simulink model "NM100A_MotVelCtrl"  (R2013b)
settings: Solver=FixedStepDiscrete  SolverMode=SingleTasking  StartTime=0.0  StopTime=1  FixedStep=0.002  RelTol=1e-3
values from neighbouring files (symbols this model uses):
  ARCHGLBPRM_2MILLISEC_SEC_F32 = DataDict.Constant    [NM100A_MotVelCtrl_DataDict.m]
  DERIVTVLPFILTICONLOWRLIM_SEC_F32 = DataDict.Constant    [NM100A_MotVelCtrl_DataDict.m]
  FALSE_CNT_LGC = DataDict.Constant    [NM100A_MotVelCtrl_DataDict.m]
  MOTVELTHDRAMPDWNCMPL_MOTRADPERSEC_F32 = DataDict.Constant    [NM100A_MotVelCtrl_DataDict.m]
  ONEMILLISEC_SEC_F32 = DataDict.Constant    [NM100A_MotVelCtrl_DataDict.m]
  TITHDRAMPDWNCMPL_CNT_U16 = DataDict.Constant    [NM100A_MotVelCtrl_DataDict.m]
  TRUE_CNT_LGC = DataDict.Constant    [NM100A_MotVelCtrl_DataDict.m]
  ZEROMOTVELTAR_MOTRADPERSEC_F32 = DataDict.Constant    [NM100A_MotVelCtrl_DataDict.m]
  ZEROTQCMD_MOTNWTMTR_F32 = DataDict.Constant    [NM100A_MotVelCtrl_DataDict.m]
libraries: NxtrLim x13, simulink x1, NxtrAbslt x1, NxtrMax x1
(part 3 of 4)

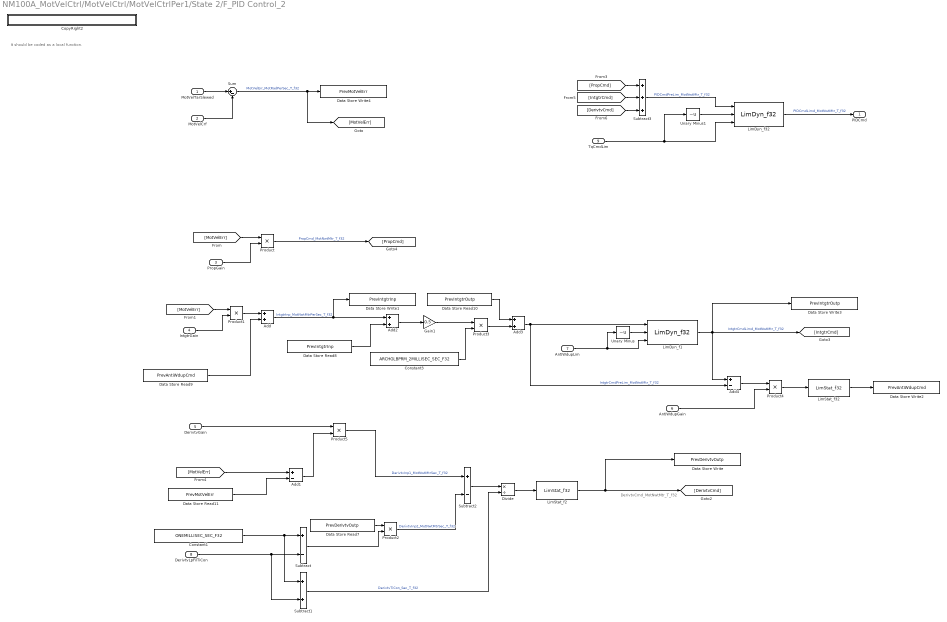
== system NM100A_MotVelCtrl/MotVelCtrl/MotVelCtrlPer1/State 2/F_PID Control_2 ==
  note: DerivtvCmd_MotNwtMtr_T_f32
  note: It should be coded as a local function.
  MotVelTarSlewed : Inport  RequirementInfo="{'linktype_rmi_doors' '00010020 (/E-STEER Core/SubSystem Specifications/Manufacturing Service/NM100A_Motor Velocity Control Function Requirement)' '#NM100A_30' 'true' 'REQ:  NM100A_30' '' } %GIDa_110524b8_0db1_43e8_8f08_01f20704c4bb"
  MotVelCrf : Inport  RequirementInfo="{'linktype_rmi_doors' '00010020 (/E-STEER Core/SubSystem Specifications/Manufacturing Service/NM100A_Motor Velocity Control Function Requirement)' '#NM100A_30' 'true' 'REQ:  NM100A_30' '' } %GIDa_7d766da7_5e04_40ea_badd_d72d93f3cd8f"  Port=2
  PropGain : Inport  RequirementInfo="{'linktype_rmi_doors' '00010020 (/E-STEER Core/SubSystem Specifications/Manufacturing Service/NM100A_Motor Velocity Control Function Requirement)' '#NM100A_112' 'true' 'REQ:  NM100A_112' '' } %GIDa_a1a22dbd_d264_4c62_8ca1_990479f3e1bd"  Port=3
  IntgtrGain : Inport  RequirementInfo="{'linktype_rmi_doors' '00010020 (/E-STEER Core/SubSystem Specifications/Manufacturing Service/NM100A_Motor Velocity Control Function Requirement)' '#NM100A_115' 'true' 'REQ:  NM100A_115' '' } %GIDa_1390f88b_fe28_4670_9b5c_e6d73974c688"  Port=4
  DerivtvGain : Inport  RequirementInfo="{'linktype_rmi_doors' '00010020 (/E-STEER Core/SubSystem Specifications/Manufacturing Service/NM100A_Motor Velocity Control Function Requirement)' '#NM100A_116' 'true' 'REQ:  NM100A_116' '' } %GIDa_f6cc3c77_9957_4476_a97a_fb14260ee4dc"  Port=5
  AntiWdupGain : Inport  RequirementInfo="{'linktype_rmi_doors' '00010020 (/E-STEER Core/SubSystem Specifications/Manufacturing Service/NM100A_Motor Velocity Control Function Requirement)' '#NM100A_118' 'true' 'REQ:  NM100A_118' '' } %GIDa_56666803_4490_41e6_aeb7_9ef0196ec25d"  Port=6
  AntiWdupLim : Inport  RequirementInfo="{'linktype_rmi_doors' '00010020 (/E-STEER Core/SubSystem Specifications/Manufacturing Service/NM100A_Motor Velocity Control Function Requirement)' '#NM100A_118' 'true' 'REQ:  NM100A_118' '' } %GIDa_11bba2b0_a075_4aca_bc0b_995865d16d8e"  Port=7
  DerivtvLpFilTiCon : Inport  RequirementInfo="{'linktype_rmi_doors' '00010020 (/E-STEER Core/SubSystem Specifications/Manufacturing Service/NM100A_Motor Velocity Control Function Requirement)' '#NM100A_116' 'true' 'REQ:  NM100A_116' '' } %GIDa_2802fec0_4346_4fda_bccf_964533d4d2f8"  Port=8
  TqCmdLim : Inport  RequirementInfo="{'linktype_rmi_doors' '00010020 (/E-STEER Core/SubSystem Specifications/Manufacturing Service/NM100A_Motor Velocity Control Function Requirement)' '#NM100A_123' 'true' 'REQ:  NM100A_123' '' } %GIDa_855cb0b5_ed49_433d_978f_0dace05c254b"  Port=9
  Add : Sum  RequirementInfo="{'linktype_rmi_doors' '00010020 (/E-STEER Core/SubSystem Specifications/Manufacturing Service/NM100A_Motor Velocity Control Function Requirement)' '#NM100A_115' 'true' 'REQ:  NM100A_115' '' } %GIDa_6815d85c_18d2_448a_90c3_eea3a5c7f45e"
  Add1 : Sum  RequirementInfo="{'linktype_rmi_doors' '00010020 (/E-STEER Core/SubSystem Specifications/Manufacturing Service/NM100A_Motor Velocity Control Function Requirement)' '#NM100A_116' 'true' 'REQ:  NM100A_116' '' } %GIDa_f4b28a13_3ee6_406c_9849_7eac37b89283"  Inputs=+-
  Add2 : Sum  RequirementInfo="{'linktype_rmi_doors' '00010020 (/E-STEER Core/SubSystem Specifications/Manufacturing Service/NM100A_Motor Velocity Control Function Requirement)' '#NM100A_115' 'true' 'REQ:  NM100A_115' '' } %GIDa_9422ee42_1d4f_4bea_b4bf_ebe76635d43d"
  Add3 : Sum  RequirementInfo="{'linktype_rmi_doors' '00010020 (/E-STEER Core/SubSystem Specifications/Manufacturing Service/NM100A_Motor Velocity Control Function Requirement)' '#NM100A_115' 'true' 'REQ:  NM100A_115' '' } %GIDa_cc936411_c916_404a_ab30_f6a397637365"
  Add4 : Sum  RequirementInfo={'linktype_rmi_doors' '00010020 (/E-STEER Core/SubSystem Specifications/Manufacturing Service/NM100A_Motor Velocity Control Function Requirement)' '#NM100A_118' 'true' 'REQ:NM100A_118' '' } %GIDa_b21f0add_36e5_418f_9ceb_17b3d59b7e90  Inputs=+-
  Constant1 : Constant  RequirementInfo="{'linktype_rmi_doors' '00010020 (/E-STEER Core/SubSystem Specifications/Manufacturing Service/NM100A_Motor Velocity Control Function Requirement)' '#NM100A_116' 'true' 'REQ:  NM100A_116' '' } %GIDa_f3e2cce3_6137_4c8a_aa56_8064cca81233"  Value=ONEMILLISEC_SEC_F32
  Constant3 : Constant  RequirementInfo="{'linktype_rmi_doors' '00010020 (/E-STEER Core/SubSystem Specifications/Manufacturing Service/NM100A_Motor Velocity Control Function Requirement)' '#NM100A_115' 'true' 'REQ:  NM100A_115' '' } %GIDa_c43bbe87_f3ae_4efd_b0d8_54889718fd03"  Value=ARCHGLBPRM_2MILLISEC_SEC_F32
  CopyRight2 : Subsystem  Description=|  mask(Copyright Information){none=on}
      | Copyright info block.                                               
      |                                                                     
      | Place copyright information at the top of every subsystem in design.
      mask prompts: none "No parameters"
      mask help: Place copyright information at the top of every subsystem in design.
      mask Display:
      | NxtrConf = 'Nexteer Confidential';
      | 
      | sys = bdroot; %handle for the current model ("system")
      | first = get_param(sys,'Created');
      | if(isempty(first))
      |     first = datestr(now,'yyyy');
      | else
      |     first = first(end-3:end);  %year is last four digits
      | end
      | 
      | last = get_param(sys,'LastModifiedDate');
      | if isempty(last)
      |     last = datestr(now,'yyyy');
      | else
      |     last = last(end-3:end);
      | end
      | 
      | if strcmp(first,last)
      |     fprintf('%s -- Copyright %s Nexteer',NxtrConf,first)
      | else
      |     fprintf('%s -- %s%s- %s Nexteer',NxtrConf,char(169),first,last)
      | end
  Data Store Read10 : DataStoreRead  RequirementInfo="{'linktype_rmi_doors' '00010020 (/E-STEER Core/SubSystem Specifications/Manufacturing Service/NM100A_Motor Velocity Control Function Requirement)' '#NM100A_115' 'true' 'REQ:  NM100A_115' '' } %GIDa_57049909_113a_42ec_bae6_d87ca5e4f12b"  Priority=1  DataStoreName=PrevIntgtrOutp
  Data Store Read11 : DataStoreRead  RequirementInfo="{'linktype_rmi_doors' '00010020 (/E-STEER Core/SubSystem Specifications/Manufacturing Service/NM100A_Motor Velocity Control Function Requirement)' '#NM100A_116' 'true' 'REQ:  NM100A_116' '' } %GIDa_9f5ca0ec_ed47_41b3_b6b4_071471159927"  Priority=1  DataStoreName=PrevMotVelErr
  Data Store Read7 : DataStoreRead  RequirementInfo="{'linktype_rmi_doors' '00010020 (/E-STEER Core/SubSystem Specifications/Manufacturing Service/NM100A_Motor Velocity Control Function Requirement)' '#NM100A_116' 'true' 'REQ:  NM100A_116' '' } %GIDa_6db4a11a_7baf_4ed8_9c4d_f159cd772cec"  Priority=1  DataStoreName=PrevDerivtvOutp
  Data Store Read8 : DataStoreRead  RequirementInfo="{'linktype_rmi_doors' '00010020 (/E-STEER Core/SubSystem Specifications/Manufacturing Service/NM100A_Motor Velocity Control Function Requirement)' '#NM100A_115' 'true' 'REQ:  NM100A_115' '' } %GIDa_7cb75691_c32e_45f7_8fbd_fb2078527a41"  Priority=1  DataStoreName=PrevIntgtrInp
  Data Store Read9 : DataStoreRead  RequirementInfo="{'linktype_rmi_doors' '00010020 (/E-STEER Core/SubSystem Specifications/Manufacturing Service/NM100A_Motor Velocity Control Function Requirement)' '#NM100A_118' 'true' 'REQ:  NM100A_118' '' } %GIDa_fca8d963_6714_4519_b1fa_d800b04f6915"  Priority=1  DataStoreName=PrevAntiWdupCmd
  Data Store Write : DataStoreWrite  RequirementInfo="{'linktype_rmi_doors' '00010020 (/E-STEER Core/SubSystem Specifications/Manufacturing Service/NM100A_Motor Velocity Control Function Requirement)' '#NM100A_116' 'true' 'REQ:  NM100A_116' '' } %GIDa_c8470beb_41bb_4bfc_8c04_56d815b5965f"  Priority=2  DataStoreName=PrevDerivtvOutp
  Data Store Write1 : DataStoreWrite  RequirementInfo="{'linktype_rmi_doors' '00010020 (/E-STEER Core/SubSystem Specifications/Manufacturing Service/NM100A_Motor Velocity Control Function Requirement)' '#NM100A_115' 'true' 'REQ:  NM100A_115' '' } %GIDa_ba0b9b43_91f2_4915_a3e9_835597968f46"  Priority=2  DataStoreName=PrevIntgtrInp
  Data Store Write2 : DataStoreWrite  RequirementInfo="{'linktype_rmi_doors' '00010020 (/E-STEER Core/SubSystem Specifications/Manufacturing Service/NM100A_Motor Velocity Control Function Requirement)' '#NM100A_118' 'true' 'REQ:  NM100A_118' '' } %GIDa_e3d6484a_1ac4_4af3_b295_acb9bb1c6154"  Priority=2  DataStoreName=PrevAntiWdupCmd
  Data Store Write3 : DataStoreWrite  RequirementInfo="{'linktype_rmi_doors' '00010020 (/E-STEER Core/SubSystem Specifications/Manufacturing Service/NM100A_Motor Velocity Control Function Requirement)' '#NM100A_115' 'true' 'REQ:  NM100A_115' '' } %GIDa_1450aec8_d417_4637_9f89_973782db30a6"  Priority=2  DataStoreName=PrevIntgtrOutp
  Data Store Write4 : DataStoreWrite  RequirementInfo="{'linktype_rmi_doors' '00010020 (/E-STEER Core/SubSystem Specifications/Manufacturing Service/NM100A_Motor Velocity Control Function Requirement)' '#NM100A_30' 'true' 'REQ:  NM100A_30' '' } %GIDa_217db27e_790d_4aff_9d20_668ede9c1fce"  Priority=2  DataStoreName=PrevMotVelErr
  Divide : Product  RequirementInfo="{'linktype_rmi_doors' '00010020 (/E-STEER Core/SubSystem Specifications/Manufacturing Service/NM100A_Motor Velocity Control Function Requirement)' '#NM100A_116' 'true' 'REQ:  NM100A_116' '' } %GIDa_54ef5091_11b4_4ec5_b890_f4b3699e9ee9"  Inputs=*/
  Gain1 : Gain  RequirementInfo="{'linktype_rmi_doors' '00010020 (/E-STEER Core/SubSystem Specifications/Manufacturing Service/NM100A_Motor Velocity Control Function Requirement)' '#NM100A_115' 'true' 'REQ:  NM100A_115' '' } %GIDa_18ede273_3183_4af6_908a_3a2887a150cf"  Gain=0.5  ParamDataTypeStr=single  OutDataTypeStr=single
  LimDyn_f1 : NxtrLim/LimDyn_f32  RequirementInfo="{'linktype_rmi_doors' '00010020 (/E-STEER Core/SubSystem Specifications/Manufacturing Service/NM100A_Motor Velocity Control Function Requirement)' '#NM100A_115' 'true' 'REQ:  NM100A_115' '' ; 'linktype_rmi_doors' '00010020 (/E-STEER Core/SubSystem Specifications/Manufacturing Service/NM100A_Motor Velocity Control Function Requirement)' '#NM100A_118' 'true' 'REQ:  NM100A_118' '' } %GIDa_98969518_5195_4cf6_a605_50c99a8888a3"
  LimDyn_f32 : NxtrLim/LimDyn_f32  RequirementInfo="{'linktype_rmi_doors' '00010020 (/E-STEER Core/SubSystem Specifications/Manufacturing Service/NM100A_Motor Velocity Control Function Requirement)' '#NM100A_123' 'true' 'REQ:  NM100A_123' '' } %GIDa_e565d932_13fb_41f6_8c00_f392cf9a5025"
  LimStat_f2 : NxtrLim/LimStat_f32  RequirementInfo={'linktype_rmi_doors' '00010020 (/E-STEER Core/SubSystem Specifications/Manufacturing Service/NM100A_Motor Velocity Control Function Requirement)' '#NM100A_116' 'true' 'REQ:NM100A_116' '' } %GIDa_c327b6ed_9cdf_449b_be36_d36427633387  LoLim=DERIVTVCMDLOWRLIM_MOTNWTMTR_F32  HiLim=DERIVTVCMDUPPRLIM_MOTNWTMTR_F32
      settings: AttributesFormatString=|
      | Low Limit: %<LoLim>
      | High Limit:%<HiLim>
  LimStat_f32 : NxtrLim/LimStat_f32  RequirementInfo={'linktype_rmi_doors' '00010020 (/E-STEER Core/SubSystem Specifications/Manufacturing Service/NM100A_Motor Velocity Control Function Requirement)' '#NM100A_118' 'true' 'REQ:NM100A_118' '' } %GIDa_a7bf9df9_073b_4216_8fa2_ddeed09f4342  LoLim=ANTIWDUPCMDLOWRLIM_MOTNWTMTR_F32  HiLim=ANTIWDUPCMDUPPRLIM_MOTNWTMTR_F32
      settings: AttributesFormatString=|
      | Low Limit: %<LoLim>
      | High Limit:%<HiLim>
  Product : Product  RequirementInfo="{'linktype_rmi_doors' '00010020 (/E-STEER Core/SubSystem Specifications/Manufacturing Service/NM100A_Motor Velocity Control Function Requirement)' '#NM100A_112' 'true' 'REQ:  NM100A_112' '' } %GIDa_8c2be680_e142_40d3_aa90_8a9abfd9ee6e"
  Product1 : Product  RequirementInfo="{'linktype_rmi_doors' '00010020 (/E-STEER Core/SubSystem Specifications/Manufacturing Service/NM100A_Motor Velocity Control Function Requirement)' '#NM100A_115' 'true' 'REQ:  NM100A_115' '' } %GIDa_69667977_5b44_4db7_8f1f_cac1dee6c049"
  Product2 : Product  RequirementInfo="{'linktype_rmi_doors' '00010020 (/E-STEER Core/SubSystem Specifications/Manufacturing Service/NM100A_Motor Velocity Control Function Requirement)' '#NM100A_116' 'true' 'REQ:  NM100A_116' '' } %GIDa_71299b77_1b0a_49c1_b0db_a584eeec07c6"
  Product3 : Product  RequirementInfo="{'linktype_rmi_doors' '00010020 (/E-STEER Core/SubSystem Specifications/Manufacturing Service/NM100A_Motor Velocity Control Function Requirement)' '#NM100A_115' 'true' 'REQ:  NM100A_115' '' } %GIDa_3f34b12f_6e4c_49db_a236_48eef5326218"
  Product4 : Product  RequirementInfo="{'linktype_rmi_doors' '00010020 (/E-STEER Core/SubSystem Specifications/Manufacturing Service/NM100A_Motor Velocity Control Function Requirement)' '#NM100A_118' 'true' 'REQ:  NM100A_118' '' } %GIDa_bdead0a2_4bcd_4088_9cb6_c5fabbc39160"
  Product5 : Product  RequirementInfo="{'linktype_rmi_doors' '00010020 (/E-STEER Core/SubSystem Specifications/Manufacturing Service/NM100A_Motor Velocity Control Function Requirement)' '#NM100A_116' 'true' 'REQ:  NM100A_116' '' } %GIDa_9bd3a447_0cd3_4969_a409_7e68280b9a84"
  Subtract : Sum  RequirementInfo="{'linktype_rmi_doors' '00010020 (/E-STEER Core/SubSystem Specifications/Manufacturing Service/NM100A_Motor Velocity Control Function Requirement)' '#NM100A_116' 'true' 'REQ:  NM100A_116' '' } %GIDa_caef336f_e7fa_4c58_ade1_c972a30702a6"  Inputs=+-
  Subtract1 : Sum  RequirementInfo="{'linktype_rmi_doors' '00010020 (/E-STEER Core/SubSystem Specifications/Manufacturing Service/NM100A_Motor Velocity Control Function Requirement)' '#NM100A_116' 'true' 'REQ:  NM100A_116' '' } %GIDa_8c405288_566e_462c_b2dc_c4bd59dc36f4"
  Subtract2 : Sum  RequirementInfo={} %GIDa_760fbade_77c6_45ff_ae65_2688be45a6f8  Inputs=+-
  Subtract3 : Sum  RequirementInfo="{'linktype_rmi_doors' '00010020 (/E-STEER Core/SubSystem Specifications/Manufacturing Service/NM100A_Motor Velocity Control Function Requirement)' '#NM100A_122' 'true' 'REQ:  NM100A_122' '' } %GIDa_ccf79976_d4cd_4874_a140_9b093bd4dd65"  Inputs=+++
  Sum : Sum  RequirementInfo="{'linktype_rmi_doors' '00010020 (/E-STEER Core/SubSystem Specifications/Manufacturing Service/NM100A_Motor Velocity Control Function Requirement)' '#NM100A_30' 'true' 'REQ:  NM100A_30' '' } %GIDa_68a72d2d_c6a4_4441_ae1b_c7e942cb1428"  Inputs=|+-
  Unary Minus : UnaryMinus  RequirementInfo="{'linktype_rmi_doors' '00010020 (/E-STEER Core/SubSystem Specifications/Manufacturing Service/NM100A_Motor Velocity Control Function Requirement)' '#NM100A_118' 'true' 'REQ:  NM100A_118' '' } %GIDa_4052e92e_b6dc_4afd_a640_75fdba6ca66d"
  Unary Minus1 : UnaryMinus  RequirementInfo="{'linktype_rmi_doors' '00010020 (/E-STEER Core/SubSystem Specifications/Manufacturing Service/NM100A_Motor Velocity Control Function Requirement)' '#NM100A_123' 'true' 'REQ:  NM100A_123' '' } %GIDa_2b0888ff_318e_4b74_8211_e2e686a97192"
  "PIDCmd " : Outport
  wires:
  [MotVelErr] -> Product/1
  PropGain/1 -> Product/2
  [MotVelErr] -> Product1/1
  IntgtrGain/1 -> Product1/2
  Product1/1 -> Add/1
  Data Store Read9/1 -> Add/2
  Add/1 -> Data Store Write1/1, Add2/1  "IntgtrInp_MotNwtMtrPerSec_T_f32"
  Add2/1 -> Gain1/1
  Gain1/1 -> Product3/1
  Constant3/1 -> Product3/2
  Product3/1 -> Add3/2
  Add3/1 -> Add4/2, LimDyn_f1/1  "IntgtrCmdPreLim_MotNwtMtr_T_f32"
  LimDyn_f1/1 -> Data Store Write3/1, Add4/1, [IntgtrCmd]  "IntgtrCmdLimd_MotNwtMtr_T_f32"
  AntiWdupLim/1 -> Unary Minus/1, LimDyn_f1/3
  Unary Minus/1 -> LimDyn_f1/2
  [MotVelErr] -> Add1/1
  Constant1/1 -> Subtract1/1, Subtract/1
  DerivtvLpFilTiCon/1 -> Subtract1/2, Subtract/2
  Subtract/1 -> Product2/2
  Data Store Read7/1 -> Product2/1
  Product2/1 -> Subtract2/2  "DerivtvInp2_MotNwtMtrSec_T_f32"
  Subtract2/1 -> Divide/1
  Subtract1/1 -> Divide/2  "DerivtvTiCon_Sec_T_f32"
  Product/1 -> [PropCmd]  "PropCmd_MotNwtMtr_T_f32"
  [PropCmd] -> Subtract3/1
  [IntgtrCmd] -> Subtract3/2
  [DerivtvCmd] -> Subtract3/3
  Subtract3/1 -> LimDyn_f32/1  "PIDCmdPreLim_MotNwtMtr_T_f32"
  Unary Minus1/1 -> LimDyn_f32/2
  TqCmdLim/1 -> LimDyn_f32/3, Unary Minus1/1
  LimDyn_f32/1 -> "PIDCmd "/1  "PIDCmdLimd_MotNwtMtr_T_f32"
  Divide/1 -> LimStat_f2/1
  Data Store Read8/1 -> Add2/2
  Data Store Read10/1 -> Add3/1
  Data Store Read11/1 -> Add1/2
  Sum/1 -> [MotVelErr], Data Store Write4/1  "MotVelErr_MotRadPerSec_T_f32"
  Add4/1 -> Product4/1
  AntiWdupGain/1 -> Product4/2
  Product4/1 -> LimStat_f32/1
  DerivtvGain/1 -> Product5/1
  Add1/1 -> Product5/2
  Product5/1 -> Subtract2/1  "DerivtvInp1_MotNwtMtrSec_T_f32"
  MotVelTarSlewed/1 -> Sum/1
  MotVelCrf/1 -> Sum/2
  LimStat_f32/1 -> Data Store Write2/1
  LimStat_f2/1 -> Data Store Write/1, [DerivtvCmd]

== system NM100A_MotVelCtrl/MotVelCtrl/MotVelCtrlPer1/State 2/GetRefTmr100MicroSec32bit ==
  note: 1 count = 100 uSec
  note: seconds
  note: microseconds
  note: counts
  note: Wrap-to-zero
  note: GetRefTmr100MicroSec32bit
  CopyRight2 : Subsystem  Description=|  mask(Copyright Information){none=on}
      | Copyright info block.                                               
      |                                                                     
      | Place copyright information at the top of every subsystem in design.
      mask prompts: none "No parameters"
      mask help: Place copyright information at the top of every subsystem in design.
      mask Display:
      | NxtrConf = 'Nexteer Confidential';
      | 
      | sys = bdroot; %handle for the current model ("system")
      | first = get_param(sys,'Created');
      | if(isempty(first))
      |     first = datestr(now,'yyyy');
      | else
      |     first = first(end-3:end);  %year is last four digits
      | end
      | 
      | last = get_param(sys,'LastModifiedDate');
      | if isempty(last)
      |     last = datestr(now,'yyyy');
      | else
      |     last = last(end-3:end);
      | end
      | 
      | if strcmp(first,last)
      |     fprintf('%s -- Copyright %s Nexteer',NxtrConf,first)
      | else
      |     fprintf('%s -- %s%s- %s Nexteer',NxtrConf,char(169),first,last)
      | end
  Count per uSec : Constant  Value=0.01
  Data Store Read1 : DataStoreRead  DataStoreName=SimnTi
  Data Type Conversion1 : DataTypeConversion  OutDataTypeStr=uint32
  Divide1 : Product  Inputs=**
  Divide2 : Product  Inputs=*/
  Max Counts : Constant  Value=2^32-1
  Product1 : Product
  Product2 : Product
  Rounding : Rounding
  Subtract1 : Sum  Inputs=+-
  uSec per Sec : Constant  Value=1000000
  RefTmr : Outport
  wires:
  Product2/1 -> Subtract1/2
  Subtract1/1 -> Data Type Conversion1/1
  Rounding/1 -> Product2/1
  Divide2/1 -> Rounding/1
  Max Counts/1 -> Divide2/2, Product2/2
  Divide1/1 -> Divide2/1, Subtract1/1
  Product1/1 -> Divide1/1
  Data Store Read1/1 -> Product1/1
  Count per uSec/1 -> Divide1/2
  uSec per Sec/1 -> Product1/2
  Data Type Conversion1/1 -> RefTmr/1

== system NM100A_MotVelCtrl/MotVelCtrl/MotVelCtrlPer1/State 2/SetManTqCmd ==
  ManTqCmd : Inport  RequirementInfo="{'linktype_rmi_doors' '00010020 (/E-STEER Core/SubSystem Specifications/Manufacturing Service/NM100A_Motor Velocity Control Function Requirement)' '#NM100A_49' 'true' 'REQ:  NM100A_49' '' } %GIDa_5843e5dc_5f94_4701_8dc4_3c675fcec53e"
  ManTqCmdEna : Inport  RequirementInfo="{'linktype_rmi_doors' '00010020 (/E-STEER Core/SubSystem Specifications/Manufacturing Service/NM100A_Motor Velocity Control Function Requirement)' '#NM100A_49' 'true' 'REQ:  NM100A_49' '' } %GIDa_3ed809a0_525c_4a48_9877_cb5f611b6774"  Port=2
  CopyRight2 : Subsystem  Description=|  mask(Copyright Information){none=on}
      | Copyright info block.                                               
      |                                                                     
      | Place copyright information at the top of every subsystem in design.
      mask prompts: none "No parameters"
      mask help: Place copyright information at the top of every subsystem in design.
      mask Display:
      | NxtrConf = 'Nexteer Confidential';
      | 
      | sys = bdroot; %handle for the current model ("system")
      | first = get_param(sys,'Created');
      | if(isempty(first))
      |     first = datestr(now,'yyyy');
      | else
      |     first = first(end-3:end);  %year is last four digits
      | end
      | 
      | last = get_param(sys,'LastModifiedDate');
      | if isempty(last)
      |     last = datestr(now,'yyyy');
      | else
      |     last = last(end-3:end);
      | end
      | 
      | if strcmp(first,last)
      |     fprintf('%s -- Copyright %s Nexteer',NxtrConf,first)
      | else
      |     fprintf('%s -- %s%s- %s Nexteer',NxtrConf,char(169),first,last)
      | end
  Data Store Write : DataStoreWrite  RequirementInfo="{'linktype_rmi_doors' '00010020 (/E-STEER Core/SubSystem Specifications/Manufacturing Service/NM100A_Motor Velocity Control Function Requirement)' '#NM100A_49' 'true' 'REQ:  NM100A_49' '' } %GIDa_ee4a940f_ece5_44c9_85e1_c53b757b1e4d"  DataStoreName=ManTqCmd
  Data Store Write1 : DataStoreWrite  RequirementInfo="{'linktype_rmi_doors' '00010020 (/E-STEER Core/SubSystem Specifications/Manufacturing Service/NM100A_Motor Velocity Control Function Requirement)' '#NM100A_49' 'true' 'REQ:  NM100A_49' '' } %GIDa_a434819a_eb4c_44a1_87fe_b48648f98d57"  DataStoreName=ManTqCmdEna
  wires:
  ManTqCmd/1 -> Data Store Write/1
  ManTqCmdEna/1 -> Data Store Write1/1

== system NM100A_MotVelCtrl/MotVelCtrl/MotVelCtrlPer1/State 3/CopyRight2 ==

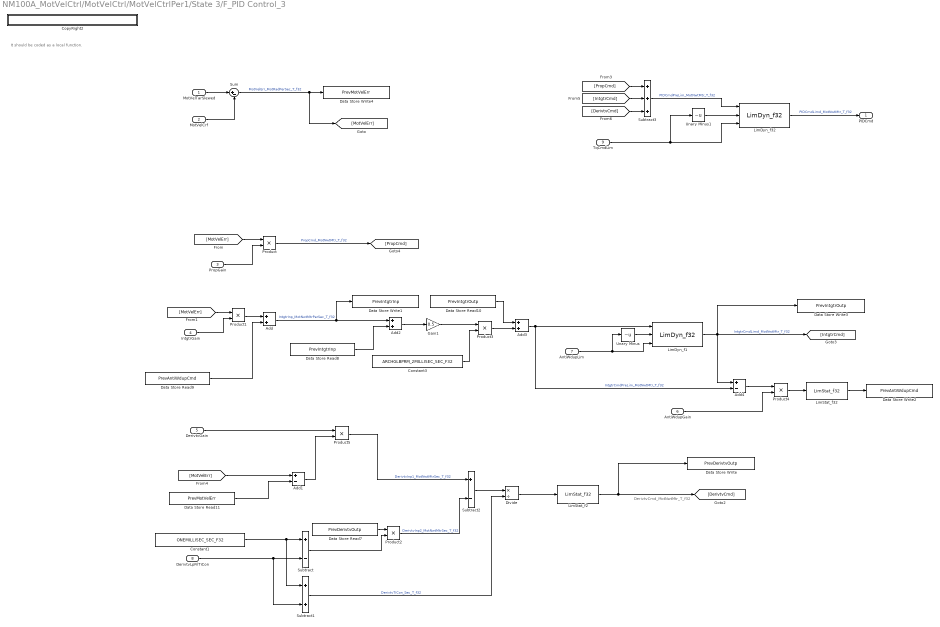
== system NM100A_MotVelCtrl/MotVelCtrl/MotVelCtrlPer1/State 3/F_PID Control_3 ==
  note: DerivtvCmd_MotNwtMtr_T_f32
  note: It should be coded as a local function.
  MotVelTarSlewed : Inport  RequirementInfo="{'linktype_rmi_doors' '00010020 (/E-STEER Core/SubSystem Specifications/Manufacturing Service/NM100A_Motor Velocity Control Function Requirement)' '#NM100A_30' 'true' 'REQ:  NM100A_30' '' } %GIDa_2385e6d7_c201_4b91_978a_d073a29ba218"
  MotVelCrf : Inport  RequirementInfo="{'linktype_rmi_doors' '00010020 (/E-STEER Core/SubSystem Specifications/Manufacturing Service/NM100A_Motor Velocity Control Function Requirement)' '#NM100A_30' 'true' 'REQ:  NM100A_30' '' } %GIDa_be6a3be8_a2c4_4431_b215_b614cdfcb56f"  Port=2
  PropGain : Inport  RequirementInfo={} %GIDa_15feff67_86e0_4f9d_b440_281f6a992387  Port=3
  IntgtrGain : Inport  RequirementInfo="{'linktype_rmi_doors' '00010020 (/E-STEER Core/SubSystem Specifications/Manufacturing Service/NM100A_Motor Velocity Control Function Requirement)' '#NM100A_115' 'true' 'REQ:  NM100A_115' '' } %GIDa_a2b014f4_d185_4d73_a152_10649d7b502b"  Port=4
  DerivtvGain : Inport  RequirementInfo="{'linktype_rmi_doors' '00010020 (/E-STEER Core/SubSystem Specifications/Manufacturing Service/NM100A_Motor Velocity Control Function Requirement)' '#NM100A_116' 'true' 'REQ:  NM100A_116' '' } %GIDa_724c960e_8de4_4ef6_90f5_ac1d7e9f190f"  Port=5
  AntiWdupGain : Inport  RequirementInfo="{'linktype_rmi_doors' '00010020 (/E-STEER Core/SubSystem Specifications/Manufacturing Service/NM100A_Motor Velocity Control Function Requirement)' '#NM100A_118' 'true' 'REQ:  NM100A_118' '' } %GIDa_41e71de3_6818_4175_9408_6c3084b80cdf"  Port=6
  AntiWdupLim : Inport  RequirementInfo="{'linktype_rmi_doors' '00010020 (/E-STEER Core/SubSystem Specifications/Manufacturing Service/NM100A_Motor Velocity Control Function Requirement)' '#NM100A_118' 'true' 'REQ:  NM100A_118' '' } %GIDa_587811f0_5d25_48e3_ba57_71c252f494bc"  Port=7
  DerivtvLpFilTiCon : Inport  RequirementInfo="{'linktype_rmi_doors' '00010020 (/E-STEER Core/SubSystem Specifications/Manufacturing Service/NM100A_Motor Velocity Control Function Requirement)' '#NM100A_116' 'true' 'REQ:  NM100A_116' '' } %GIDa_3b2f4540_a96c_494d_925d_4c1cf4c6bc80"  Port=8
  TqCmdLim : Inport  RequirementInfo="{'linktype_rmi_doors' '00010020 (/E-STEER Core/SubSystem Specifications/Manufacturing Service/NM100A_Motor Velocity Control Function Requirement)' '#NM100A_123' 'true' 'REQ:  NM100A_123' '' } %GIDa_50b7e518_24ea_4964_b8e7_0f66db1f80b4"  Port=9
  Add : Sum  RequirementInfo="{'linktype_rmi_doors' '00010020 (/E-STEER Core/SubSystem Specifications/Manufacturing Service/NM100A_Motor Velocity Control Function Requirement)' '#NM100A_115' 'true' 'REQ:  NM100A_115' '' } %GIDa_57c093c7_8a13_4742_87e5_fd49ecaf1019"
  Add1 : Sum  RequirementInfo="{'linktype_rmi_doors' '00010020 (/E-STEER Core/SubSystem Specifications/Manufacturing Service/NM100A_Motor Velocity Control Function Requirement)' '#NM100A_116' 'true' 'REQ:  NM100A_116' '' } %GIDa_564ff11f_e14e_4f44_888d_2792856171ea"  Inputs=+-
  Add2 : Sum  RequirementInfo="{'linktype_rmi_doors' '00010020 (/E-STEER Core/SubSystem Specifications/Manufacturing Service/NM100A_Motor Velocity Control Function Requirement)' '#NM100A_115' 'true' 'REQ:  NM100A_115' '' } %GIDa_6259ee55_4b71_4607_8b54_6ac4d4862bb5"
  Add3 : Sum  RequirementInfo="{'linktype_rmi_doors' '00010020 (/E-STEER Core/SubSystem Specifications/Manufacturing Service/NM100A_Motor Velocity Control Function Requirement)' '#NM100A_115' 'true' 'REQ:  NM100A_115' '' } %GIDa_ac2428de_b1a3_4fef_8682_d84eab9256f7"
  Add4 : Sum  RequirementInfo={'linktype_rmi_doors' '00010020 (/E-STEER Core/SubSystem Specifications/Manufacturing Service/NM100A_Motor Velocity Control Function Requirement)' '#NM100A_118' 'true' 'REQ:NM100A_118' '' } %GIDa_7578dfa8_5d6d_426e_8eb1_c4aa91a9f3e9  Inputs=+-
  Constant1 : Constant  RequirementInfo="{'linktype_rmi_doors' '00010020 (/E-STEER Core/SubSystem Specifications/Manufacturing Service/NM100A_Motor Velocity Control Function Requirement)' '#NM100A_116' 'true' 'REQ:  NM100A_116' '' } %GIDa_16546e68_ed3d_431c_b147_f8aa2ac02bc5"  Value=ONEMILLISEC_SEC_F32
  Constant3 : Constant  RequirementInfo="{'linktype_rmi_doors' '00010020 (/E-STEER Core/SubSystem Specifications/Manufacturing Service/NM100A_Motor Velocity Control Function Requirement)' '#NM100A_115' 'true' 'REQ:  NM100A_115' '' } %GIDa_5813c373_d203_49ef_b653_63bc4179cd37"  Value=ARCHGLBPRM_2MILLISEC_SEC_F32
  CopyRight2 : Subsystem  Description=|  mask(Copyright Information){none=on}
      | Copyright info block.                                               
      |                                                                     
      | Place copyright information at the top of every subsystem in design.
      mask prompts: none "No parameters"
      mask help: Place copyright information at the top of every subsystem in design.
      mask Display:
      | NxtrConf = 'Nexteer Confidential';
      | 
      | sys = bdroot; %handle for the current model ("system")
      | first = get_param(sys,'Created');
      | if(isempty(first))
      |     first = datestr(now,'yyyy');
      | else
      |     first = first(end-3:end);  %year is last four digits
      | end
      | 
      | last = get_param(sys,'LastModifiedDate');
      | if isempty(last)
      |     last = datestr(now,'yyyy');
      | else
      |     last = last(end-3:end);
      | end
      | 
      | if strcmp(first,last)
      |     fprintf('%s -- Copyright %s Nexteer',NxtrConf,first)
      | else
      |     fprintf('%s -- %s%s- %s Nexteer',NxtrConf,char(169),first,last)
      | end
  Data Store Read10 : DataStoreRead  RequirementInfo="{'linktype_rmi_doors' '00010020 (/E-STEER Core/SubSystem Specifications/Manufacturing Service/NM100A_Motor Velocity Control Function Requirement)' '#NM100A_115' 'true' 'REQ:  NM100A_115' '' } %GIDa_f673c82f_04fa_4bcf_a953_d7351d447037"  Priority=1  DataStoreName=PrevIntgtrOutp
  Data Store Read11 : DataStoreRead  RequirementInfo="{'linktype_rmi_doors' '00010020 (/E-STEER Core/SubSystem Specifications/Manufacturing Service/NM100A_Motor Velocity Control Function Requirement)' '#NM100A_116' 'true' 'REQ:  NM100A_116' '' } %GIDa_e5fb83f9_a74f_4aef_a092_6f7aeafb88b8"  Priority=1  DataStoreName=PrevMotVelErr
  Data Store Read7 : DataStoreRead  RequirementInfo="{'linktype_rmi_doors' '00010020 (/E-STEER Core/SubSystem Specifications/Manufacturing Service/NM100A_Motor Velocity Control Function Requirement)' '#NM100A_116' 'true' 'REQ:  NM100A_116' '' } %GIDa_13a3d8fd_d92d_4b33_8a6e_b2babca3cb6b"  Priority=1  DataStoreName=PrevDerivtvOutp
  Data Store Read8 : DataStoreRead  RequirementInfo="{'linktype_rmi_doors' '00010020 (/E-STEER Core/SubSystem Specifications/Manufacturing Service/NM100A_Motor Velocity Control Function Requirement)' '#NM100A_115' 'true' 'REQ:  NM100A_115' '' } %GIDa_42cdca1b_edde_456c_90f5_542a7b0c2f3a"  Priority=1  DataStoreName=PrevIntgtrInp
  Data Store Read9 : DataStoreRead  RequirementInfo="{'linktype_rmi_doors' '00010020 (/E-STEER Core/SubSystem Specifications/Manufacturing Service/NM100A_Motor Velocity Control Function Requirement)' '#NM100A_118' 'true' 'REQ:  NM100A_118' '' } %GIDa_7a9924a4_a50a_486f_8642_12f74570fb29"  Priority=1  DataStoreName=PrevAntiWdupCmd
  Data Store Write : DataStoreWrite  RequirementInfo="{'linktype_rmi_doors' '00010020 (/E-STEER Core/SubSystem Specifications/Manufacturing Service/NM100A_Motor Velocity Control Function Requirement)' '#NM100A_116' 'true' 'REQ:  NM100A_116' '' } %GIDa_065bb572_d774_4474_8d90_5bd182c6c858"  Priority=2  DataStoreName=PrevDerivtvOutp
  Data Store Write1 : DataStoreWrite  RequirementInfo="{'linktype_rmi_doors' '00010020 (/E-STEER Core/SubSystem Specifications/Manufacturing Service/NM100A_Motor Velocity Control Function Requirement)' '#NM100A_115' 'true' 'REQ:  NM100A_115' '' } %GIDa_06483eec_b65f_43a6_928f_d115e935b2b1"  Priority=2  DataStoreName=PrevIntgtrInp
  Data Store Write2 : DataStoreWrite  RequirementInfo="{'linktype_rmi_doors' '00010020 (/E-STEER Core/SubSystem Specifications/Manufacturing Service/NM100A_Motor Velocity Control Function Requirement)' '#NM100A_118' 'true' 'REQ:  NM100A_118' '' } %GIDa_dc87af62_bf85_4620_b749_7993c340aca4"  Priority=2  DataStoreName=PrevAntiWdupCmd
  Data Store Write3 : DataStoreWrite  RequirementInfo="{'linktype_rmi_doors' '00010020 (/E-STEER Core/SubSystem Specifications/Manufacturing Service/NM100A_Motor Velocity Control Function Requirement)' '#NM100A_115' 'true' 'REQ:  NM100A_115' '' } %GIDa_2af9f55d_0c1f_470e_9f53_6d73bfe565d7"  Priority=2  DataStoreName=PrevIntgtrOutp
  Data Store Write4 : DataStoreWrite  RequirementInfo="{'linktype_rmi_doors' '00010020 (/E-STEER Core/SubSystem Specifications/Manufacturing Service/NM100A_Motor Velocity Control Function Requirement)' '#NM100A_30' 'true' 'REQ:  NM100A_30' '' } %GIDa_de65d6b7_def5_478c_b4be_094ca97e8d74"  Priority=2  DataStoreName=PrevMotVelErr
  Divide : Product  RequirementInfo="{'linktype_rmi_doors' '00010020 (/E-STEER Core/SubSystem Specifications/Manufacturing Service/NM100A_Motor Velocity Control Function Requirement)' '#NM100A_116' 'true' 'REQ:  NM100A_116' '' } %GIDa_01227a99_0aa6_449c_a0e1_fd354996cf91"  Inputs=*/
  Gain1 : Gain  RequirementInfo="{'linktype_rmi_doors' '00010020 (/E-STEER Core/SubSystem Specifications/Manufacturing Service/NM100A_Motor Velocity Control Function Requirement)' '#NM100A_115' 'true' 'REQ:  NM100A_115' '' } %GIDa_8d700aa5_141c_465e_9a31_01791b7aa31e"  Gain=0.5  ParamDataTypeStr=single  OutDataTypeStr=single
  LimDyn_f1 : NxtrLim/LimDyn_f32  RequirementInfo="{'linktype_rmi_doors' '00010020 (/E-STEER Core/SubSystem Specifications/Manufacturing Service/NM100A_Motor Velocity Control Function Requirement)' '#NM100A_115' 'true' 'REQ:  NM100A_115' '' ; 'linktype_rmi_doors' '00010020 (/E-STEER Core/SubSystem Specifications/Manufacturing Service/NM100A_Motor Velocity Control Function Requirement)' '#NM100A_118' 'true' 'REQ:  NM100A_118' '' } %GIDa_9b052462_6c77_4179_8839_45cadcd66bc4"
  LimDyn_f32 : NxtrLim/LimDyn_f32  RequirementInfo="{'linktype_rmi_doors' '00010020 (/E-STEER Core/SubSystem Specifications/Manufacturing Service/NM100A_Motor Velocity Control Function Requirement)' '#NM100A_123' 'true' 'REQ:  NM100A_123' '' } %GIDa_e55a4273_3c45_476e_b3d7_6d1039572013"
  LimStat_f2 : NxtrLim/LimStat_f32  RequirementInfo={'linktype_rmi_doors' '00010020 (/E-STEER Core/SubSystem Specifications/Manufacturing Service/NM100A_Motor Velocity Control Function Requirement)' '#NM100A_116' 'true' 'REQ:NM100A_116' '' } %GIDa_0cfd5bac_22cb_46f6_a19e_4d2d8a2ef0be  LoLim=DERIVTVCMDLOWRLIM_MOTNWTMTR_F32  HiLim=DERIVTVCMDUPPRLIM_MOTNWTMTR_F32
      settings: AttributesFormatString=|
      | Low Limit: %<LoLim>
      | High Limit:%<HiLim>
  LimStat_f32 : NxtrLim/LimStat_f32  RequirementInfo={'linktype_rmi_doors' '00010020 (/E-STEER Core/SubSystem Specifications/Manufacturing Service/NM100A_Motor Velocity Control Function Requirement)' '#NM100A_118' 'true' 'REQ:NM100A_118' '' } %GIDa_f2369cd6_e3ac_4e9b_b9f2_2fdba1705c9d  LoLim=ANTIWDUPCMDLOWRLIM_MOTNWTMTR_F32  HiLim=ANTIWDUPCMDUPPRLIM_MOTNWTMTR_F32
      settings: AttributesFormatString=|
      | Low Limit: %<LoLim>
      | High Limit:%<HiLim>
  Product : Product  RequirementInfo="{'linktype_rmi_doors' '00010020 (/E-STEER Core/SubSystem Specifications/Manufacturing Service/NM100A_Motor Velocity Control Function Requirement)' '#NM100A_112' 'true' 'REQ:  NM100A_112' '' } %GIDa_8be1b149_8b08_4d3c_ada5_d6d3ad0681b3"
  Product1 : Product  RequirementInfo="{'linktype_rmi_doors' '00010020 (/E-STEER Core/SubSystem Specifications/Manufacturing Service/NM100A_Motor Velocity Control Function Requirement)' '#NM100A_115' 'true' 'REQ:  NM100A_115' '' } %GIDa_4fb0a520_ee39_403e_aa31_835fedc65637"
  Product2 : Product  RequirementInfo="{'linktype_rmi_doors' '00010020 (/E-STEER Core/SubSystem Specifications/Manufacturing Service/NM100A_Motor Velocity Control Function Requirement)' '#NM100A_116' 'true' 'REQ:  NM100A_116' '' } %GIDa_e6df1d57_e1dc_458a_9e8c_401b50b7d320"
  Product3 : Product  RequirementInfo="{'linktype_rmi_doors' '00010020 (/E-STEER Core/SubSystem Specifications/Manufacturing Service/NM100A_Motor Velocity Control Function Requirement)' '#NM100A_115' 'true' 'REQ:  NM100A_115' '' } %GIDa_8434cd62_8e93_4d19_af1e_20770a3ae6ef"
  Product4 : Product  RequirementInfo="{'linktype_rmi_doors' '00010020 (/E-STEER Core/SubSystem Specifications/Manufacturing Service/NM100A_Motor Velocity Control Function Requirement)' '#NM100A_118' 'true' 'REQ:  NM100A_118' '' } %GIDa_8fd803b8_69ad_4949_87bf_533091e819f9"
  Product5 : Product  RequirementInfo="{'linktype_rmi_doors' '00010020 (/E-STEER Core/SubSystem Specifications/Manufacturing Service/NM100A_Motor Velocity Control Function Requirement)' '#NM100A_116' 'true' 'REQ:  NM100A_116' '' } %GIDa_385fa933_274c_4476_9823_72106ad63e91"
  Subtract : Sum  RequirementInfo="{'linktype_rmi_doors' '00010020 (/E-STEER Core/SubSystem Specifications/Manufacturing Service/NM100A_Motor Velocity Control Function Requirement)' '#NM100A_116' 'true' 'REQ:  NM100A_116' '' } %GIDa_a814af7e_35d8_4ac0_ac6d_53274c027d7f"  Inputs=+-
  Subtract1 : Sum  RequirementInfo="{'linktype_rmi_doors' '00010020 (/E-STEER Core/SubSystem Specifications/Manufacturing Service/NM100A_Motor Velocity Control Function Requirement)' '#NM100A_116' 'true' 'REQ:  NM100A_116' '' } %GIDa_3980c670_73a5_45f3_bdb8_58ea2ea24096"
  Subtract2 : Sum  RequirementInfo="{'linktype_rmi_doors' '00010020 (/E-STEER Core/SubSystem Specifications/Manufacturing Service/NM100A_Motor Velocity Control Function Requirement)' '#NM100A_116' 'true' 'REQ:  NM100A_116' '' } %GIDa_3227fe40_52bd_44c2_944b_80dcae19ebdc"  Inputs=+-
  Subtract3 : Sum  RequirementInfo="{'linktype_rmi_doors' '00010020 (/E-STEER Core/SubSystem Specifications/Manufacturing Service/NM100A_Motor Velocity Control Function Requirement)' '#NM100A_122' 'true' 'REQ:  NM100A_122' '' } %GIDa_506f1ab1_7dcb_4ccd_9509_579f24194455"  Inputs=+++
  Sum : Sum  RequirementInfo="{'linktype_rmi_doors' '00010020 (/E-STEER Core/SubSystem Specifications/Manufacturing Service/NM100A_Motor Velocity Control Function Requirement)' '#NM100A_30' 'true' 'REQ:  NM100A_30' '' } %GIDa_5f65ff37_8f73_4bc0_94cb_167ab04a15a6"  Inputs=|+-
  Unary Minus : UnaryMinus  RequirementInfo="{'linktype_rmi_doors' '00010020 (/E-STEER Core/SubSystem Specifications/Manufacturing Service/NM100A_Motor Velocity Control Function Requirement)' '#NM100A_118' 'true' 'REQ:  NM100A_118' '' } %GIDa_c250f5bf_643e_43ff_821e_199a8e61bf03"
  Unary Minus1 : UnaryMinus  RequirementInfo="{'linktype_rmi_doors' '00010020 (/E-STEER Core/SubSystem Specifications/Manufacturing Service/NM100A_Motor Velocity Control Function Requirement)' '#NM100A_123' 'true' 'REQ:  NM100A_123' '' } %GIDa_da58cd3e_21af_485a_aa7b_ad82fd7cd03a"
  "PIDCmd " : Outport
  wires:
  [MotVelErr] -> Product/1
  PropGain/1 -> Product/2
  [MotVelErr] -> Product1/1
  IntgtrGain/1 -> Product1/2
  Product1/1 -> Add/1
  Data Store Read9/1 -> Add/2
  Add/1 -> Data Store Write1/1, Add2/1  "IntgtrInp_MotNwtMtrPerSec_T_f32"
  Add2/1 -> Gain1/1
  Gain1/1 -> Product3/1
  Constant3/1 -> Product3/2
  Product3/1 -> Add3/2
  Add3/1 -> Add4/2, LimDyn_f1/1  "IntgtrCmdPreLim_MotNwtMtr_T_f32"
  LimDyn_f1/1 -> Data Store Write3/1, Add4/1, [IntgtrCmd]  "IntgtrCmdLimd_MotNwtMtr_T_f32"
  AntiWdupLim/1 -> Unary Minus/1, LimDyn_f1/3
  Unary Minus/1 -> LimDyn_f1/2
  [MotVelErr] -> Add1/1
  Constant1/1 -> Subtract1/1, Subtract/1
  DerivtvLpFilTiCon/1 -> Subtract1/2, Subtract/2
  Subtract/1 -> Product2/2
  Data Store Read7/1 -> Product2/1
  Product2/1 -> Subtract2/2  "DerivtvInp2_MotNwtMtrSec_T_f32"
  Subtract2/1 -> Divide/1
  Subtract1/1 -> Divide/2  "DerivtvTiCon_Sec_T_f32"
  Product/1 -> [PropCmd]  "PropCmd_MotNwtMtr_T_f32"
  [PropCmd] -> Subtract3/1
  [IntgtrCmd] -> Subtract3/2
  [DerivtvCmd] -> Subtract3/3
  Subtract3/1 -> LimDyn_f32/1  "PIDCmdPreLim_MotNwtMtr_T_f32"
  Unary Minus1/1 -> LimDyn_f32/2
  TqCmdLim/1 -> LimDyn_f32/3, Unary Minus1/1
  LimDyn_f32/1 -> "PIDCmd "/1  "PIDCmdLimd_MotNwtMtr_T_f32"
  Divide/1 -> LimStat_f2/1
  Data Store Read8/1 -> Add2/2
  Data Store Read10/1 -> Add3/1
  Data Store Read11/1 -> Add1/2
  Sum/1 -> [MotVelErr], Data Store Write4/1  "MotVelErr_MotRadPerSec_T_f32"
  Add4/1 -> Product4/1
  AntiWdupGain/1 -> Product4/2
  Product4/1 -> LimStat_f32/1
  DerivtvGain/1 -> Product5/1
  Add1/1 -> Product5/2
  Product5/1 -> Subtract2/1  "DerivtvInp1_MotNwtMtrSec_T_f32"
  MotVelTarSlewed/1 -> Sum/1
  MotVelCrf/1 -> Sum/2
  LimStat_f32/1 -> Data Store Write2/1
  LimStat_f2/1 -> Data Store Write/1, [DerivtvCmd]

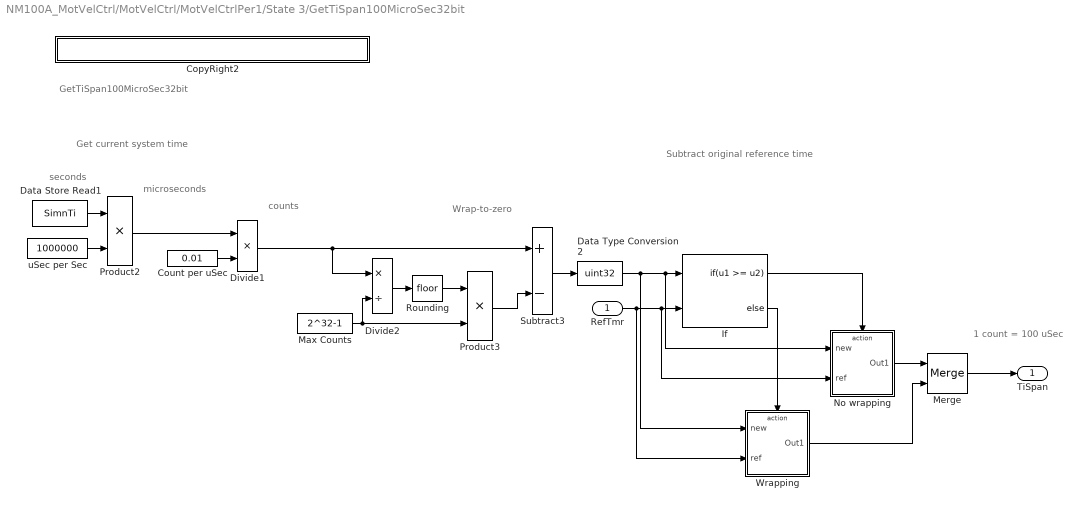
== system NM100A_MotVelCtrl/MotVelCtrl/MotVelCtrlPer1/State 3/GetTiSpan100MicroSec32bit ==
  note: Subtract original reference time
  note: seconds
  note: microseconds
  note: counts
  note: Wrap-to-zero
  note: 1 count = 100 uSec
  note: Get current system time
  note: GetTiSpan100MicroSec32bit
  RefTmr : Inport
  CopyRight2 : Subsystem  Description=|  mask(Copyright Information){none=on}
      | Copyright info block.                                               
      |                                                                     
      | Place copyright information at the top of every subsystem in design.
      mask prompts: none "No parameters"
      mask help: Place copyright information at the top of every subsystem in design.
      mask Display:
      | NxtrConf = 'Nexteer Confidential';
      | 
      | sys = bdroot; %handle for the current model ("system")
      | first = get_param(sys,'Created');
      | if(isempty(first))
      |     first = datestr(now,'yyyy');
      | else
      |     first = first(end-3:end);  %year is last four digits
      | end
      | 
      | last = get_param(sys,'LastModifiedDate');
      | if isempty(last)
      |     last = datestr(now,'yyyy');
      | else
      |     last = last(end-3:end);
      | end
      | 
      | if strcmp(first,last)
      |     fprintf('%s -- Copyright %s Nexteer',NxtrConf,first)
      | else
      |     fprintf('%s -- %s%s- %s Nexteer',NxtrConf,char(169),first,last)
      | end
  Count per uSec : Constant  Value=0.01
  Data Store Read1 : DataStoreRead  DataStoreName=SimnTi
  Data Type Conversion2 : DataTypeConversion  OutDataTypeStr=uint32
  Divide1 : Product  Inputs=**
  Divide2 : Product  Inputs=*/
  If : If  NumInputs=2  IfExpression=u1 >= u2
  Max Counts : Constant  Value=2^32-1
  Merge : Merge
  No wrapping : Subsystem  TreatAsAtomicUnit=on
  Product2 : Product
  Product3 : Product
  Rounding : Rounding
  Subtract3 : Sum  Inputs=+-
  Wrapping : Subsystem  TreatAsAtomicUnit=on
  uSec per Sec : Constant  Value=1000000
  TiSpan : Outport
  wires:
  Wrapping/1(Out1) -> Merge/2
  No wrapping/1(Out1) -> Merge/1
  If/2 -> Wrapping/Action
  If/1 -> No wrapping/Action
  Product3/1 -> Subtract3/2
  Subtract3/1 -> Data Type Conversion2/1
  Rounding/1 -> Product3/1
  Divide2/1 -> Rounding/1
  Max Counts/1 -> Divide2/2, Product3/2
  Divide1/1 -> Divide2/1, Subtract3/1
  Product2/1 -> Divide1/1
  Data Store Read1/1 -> Product2/1
  Count per uSec/1 -> Divide1/2
  uSec per Sec/1 -> Product2/2
  Merge/1 -> TiSpan/1
  RefTmr/1 -> If/2, No wrapping/2(ref), Wrapping/2(ref)
  Data Type Conversion2/1 -> If/1, No wrapping/1(new), Wrapping/1(new)

== system NM100A_MotVelCtrl/MotVelCtrl/MotVelCtrlPer1/State 3/If Action Subsystem ==
  Action Port : ActionPort  ActionType=then
  Constant1 : Constant  RequirementInfo="{'linktype_rmi_doors' '00010020 (/E-STEER Core/SubSystem Specifications/Manufacturing Service/NM100A_Motor Velocity Control Function Requirement)' '#NM100A_102' 'true' 'REQ:  NM100A_102' '' } %GIDa_6d2f279d_36df_4262_bb1b_de1400885af3"  Value=TRUE_CNT_LGC
  CopyRight2 : Subsystem  Description=|  mask(Copyright Information){none=on}
      | Copyright info block.                                               
      |                                                                     
      | Place copyright information at the top of every subsystem in design.
      mask prompts: none "No parameters"
      mask help: Place copyright information at the top of every subsystem in design.
      mask Display:
      | NxtrConf = 'Nexteer Confidential';
      | 
      | sys = bdroot; %handle for the current model ("system")
      | first = get_param(sys,'Created');
      | if(isempty(first))
      |     first = datestr(now,'yyyy');
      | else
      |     first = first(end-3:end);  %year is last four digits
      | end
      | 
      | last = get_param(sys,'LastModifiedDate');
      | if isempty(last)
      |     last = datestr(now,'yyyy');
      | else
      |     last = last(end-3:end);
      | end
      | 
      | if strcmp(first,last)
      |     fprintf('%s -- Copyright %s Nexteer',NxtrConf,first)
      | else
      |     fprintf('%s -- %s%s- %s Nexteer',NxtrConf,char(169),first,last)
      | end
  Data Store Write2 : DataStoreWrite  RequirementInfo="{'linktype_rmi_doors' '00010020 (/E-STEER Core/SubSystem Specifications/Manufacturing Service/NM100A_Motor Velocity Control Function Requirement)' '#NM100A_102' 'true' 'REQ:  NM100A_102' '' } %GIDa_b6d2c545_34e2_4d7e_8271_c5155b47dee5"  DataStoreName=RampDwnCmpl
  wires:
  Constant1/1 -> Data Store Write2/1

== system NM100A_MotVelCtrl/MotVelCtrl/MotVelCtrlPer1/State 3/SetManTqCmd ==
  ManTqCmd : Inport  RequirementInfo="{'linktype_rmi_doors' '00010020 (/E-STEER Core/SubSystem Specifications/Manufacturing Service/NM100A_Motor Velocity Control Function Requirement)' '#NM100A_51' 'true' 'REQ:  NM100A_51' '' } %GIDa_5966e690_1465_4fba_abd9_f6dae2d000c7"
  ManTqCmdEna : Inport  RequirementInfo="{'linktype_rmi_doors' '00010020 (/E-STEER Core/SubSystem Specifications/Manufacturing Service/NM100A_Motor Velocity Control Function Requirement)' '#NM100A_51' 'true' 'REQ:  NM100A_51' '' } %GIDa_b0aff816_5720_4562_8878_3df20a41f426"  Port=2
  CopyRight2 : Subsystem  Description=|  mask(Copyright Information){none=on}
      | Copyright info block.                                               
      |                                                                     
      | Place copyright information at the top of every subsystem in design.
      mask prompts: none "No parameters"
      mask help: Place copyright information at the top of every subsystem in design.
      mask Display:
      | NxtrConf = 'Nexteer Confidential';
      | 
      | sys = bdroot; %handle for the current model ("system")
      | first = get_param(sys,'Created');
      | if(isempty(first))
      |     first = datestr(now,'yyyy');
      | else
      |     first = first(end-3:end);  %year is last four digits
      | end
      | 
      | last = get_param(sys,'LastModifiedDate');
      | if isempty(last)
      |     last = datestr(now,'yyyy');
      | else
      |     last = last(end-3:end);
      | end
      | 
      | if strcmp(first,last)
      |     fprintf('%s -- Copyright %s Nexteer',NxtrConf,first)
      | else
      |     fprintf('%s -- %s%s- %s Nexteer',NxtrConf,char(169),first,last)
      | end
  Data Store Write : DataStoreWrite  RequirementInfo="{'linktype_rmi_doors' '00010020 (/E-STEER Core/SubSystem Specifications/Manufacturing Service/NM100A_Motor Velocity Control Function Requirement)' '#NM100A_51' 'true' 'REQ:  NM100A_51' '' } %GIDa_78379676_a46d_4b81_84f8_ccea39771718"  DataStoreName=ManTqCmd
  Data Store Write1 : DataStoreWrite  RequirementInfo="{'linktype_rmi_doors' '00010020 (/E-STEER Core/SubSystem Specifications/Manufacturing Service/NM100A_Motor Velocity Control Function Requirement)' '#NM100A_51' 'true' 'REQ:  NM100A_51' '' } %GIDa_ec959456_9b0a_4770_82a8_3394c3623016"  DataStoreName=ManTqCmdEna
  wires:
  ManTqCmd/1 -> Data Store Write/1
  ManTqCmdEna/1 -> Data Store Write1/1

== system NM100A_MotVelCtrl/MotVelCtrl/MotVelCtrlPer1/State 4/CopyRight2 ==

== system NM100A_MotVelCtrl/MotVelCtrl/MotVelCtrlPer1/State 4/SetManTqCmd ==
  ManTqCmd : Inport  RequirementInfo="{'linktype_rmi_doors' '00010020 (/E-STEER Core/SubSystem Specifications/Manufacturing Service/NM100A_Motor Velocity Control Function Requirement)' '#NM100A_103' 'true' 'REQ:  NM100A_103' '' } %GIDa_a9f23339_5bad_4b0b_bf0d_bc7e3a54b184"
  ManTqCmdEna : Inport  RequirementInfo="{'linktype_rmi_doors' '00010020 (/E-STEER Core/SubSystem Specifications/Manufacturing Service/NM100A_Motor Velocity Control Function Requirement)' '#NM100A_103' 'true' 'REQ:  NM100A_103' '' } %GIDa_39678411_3bd4_46d9_9a96_c987b8487f2d"  Port=2
  CopyRight2 : Subsystem  Description=|  mask(Copyright Information){none=on}
      | Copyright info block.                                               
      |                                                                     
      | Place copyright information at the top of every subsystem in design.
      mask prompts: none "No parameters"
      mask help: Place copyright information at the top of every subsystem in design.
      mask Display:
      | NxtrConf = 'Nexteer Confidential';
      | 
      | sys = bdroot; %handle for the current model ("system")
      | first = get_param(sys,'Created');
      | if(isempty(first))
      |     first = datestr(now,'yyyy');
      | else
      |     first = first(end-3:end);  %year is last four digits
      | end
      | 
      | last = get_param(sys,'LastModifiedDate');
      | if isempty(last)
      |     last = datestr(now,'yyyy');
      | else
      |     last = last(end-3:end);
      | end
      | 
      | if strcmp(first,last)
      |     fprintf('%s -- Copyright %s Nexteer',NxtrConf,first)
      | else
      |     fprintf('%s -- %s%s- %s Nexteer',NxtrConf,char(169),first,last)
      | end
  Data Store Write : DataStoreWrite  RequirementInfo="{'linktype_rmi_doors' '00010020 (/E-STEER Core/SubSystem Specifications/Manufacturing Service/NM100A_Motor Velocity Control Function Requirement)' '#NM100A_103' 'true' 'REQ:  NM100A_103' '' } %GIDa_ccdd2248_ae70_4678_974f_0579ec45f3e7"  DataStoreName=ManTqCmd
  Data Store Write1 : DataStoreWrite  RequirementInfo="{'linktype_rmi_doors' '00010020 (/E-STEER Core/SubSystem Specifications/Manufacturing Service/NM100A_Motor Velocity Control Function Requirement)' '#NM100A_103' 'true' 'REQ:  NM100A_103' '' } %GIDa_0f28ca15_6284_4e39_b71b_37e4e4e5a05c"  DataStoreName=ManTqCmdEna
  wires:
  ManTqCmd/1 -> Data Store Write/1
  ManTqCmdEna/1 -> Data Store Write1/1

== system NM100A_MotVelCtrl/MotVelCtrl/MotVelCtrlPer1/State 5 Do Nothing/CopyRight2 ==

== system NM100A_MotVelCtrl/MotVelCtrl/MotVelCtrlPer1/State 1/F_PID Control_1/CopyRight2 ==

== system NM100A_MotVelCtrl/MotVelCtrl/MotVelCtrlPer1/State 1/SetManTqCmd/CopyRight2 ==

== system NM100A_MotVelCtrl/MotVelCtrl/MotVelCtrlPer1/State 2/F_PID Control_2/CopyRight2 ==

== system NM100A_MotVelCtrl/MotVelCtrl/MotVelCtrlPer1/State 2/GetRefTmr100MicroSec32bit/CopyRight2 ==

== system NM100A_MotVelCtrl/MotVelCtrl/MotVelCtrlPer1/State 2/SetManTqCmd/CopyRight2 ==

== system NM100A_MotVelCtrl/MotVelCtrl/MotVelCtrlPer1/State 3/F_PID Control_3/CopyRight2 ==

== system NM100A_MotVelCtrl/MotVelCtrl/MotVelCtrlPer1/State 3/GetTiSpan100MicroSec32bit/CopyRight2 ==

== system NM100A_MotVelCtrl/MotVelCtrl/MotVelCtrlPer1/State 3/GetTiSpan100MicroSec32bit/No wrapping ==
  new : Inport
  ref : Inport  Port=2
  Action Port : ActionPort  ActionType=then
  Subtract1 : Sum  Inputs=+-
  Out1 : Outport
  wires:
  ref/1 -> Subtract1/2
  new/1 -> Subtract1/1
  Subtract1/1 -> Out1/1
